simulink model "NewSim"  (R2016b)
settings: Solver=ode4  StartTime=0.0  StopTime=duration  FixedStep=t_step  RelTol=1e-3
values from neighbouring files (symbols this model uses):
  albedo = [0	0.367	0.12	0.15	0.06]'    [SimSetup.m]
  constants = [6.67408e-11; 299792458; 1361; 1.38064852e-23]    [SimSetup.m]
  Cyc_pos0 = Cyc_pos0*149597870.700e3    [SimSetup.m]
  Cyc_vel0 = Cyc_vel0*149597870.700e3/86400.0    [SimSetup.m]
  desired_trajectory = desired_trajectory*149597870.700e3    [SimSetup.m]
  dim = [6;30]    [SimSetup.m]
  emis = [0 0.9 0.9 0.8 0.93]'    [SimSetup.m]
  Ki = 1e-12    [SimSetup.m]
  Kp = 1e-3    (= 0.001)    [SimSetup.m]
  mass = [1.9885E+30	5.9722E+24	7.3490E+22	6.4171E+23	1.0800E+16,250000]'    [SimSetup.m]
  radii = [695700 6378.137 1737.53 3389.92 11.16666667]'    [SimSetup.m]
  SPM_pos0 = SPM_pos0*149597870.700e3    [SimSetup.m]
  SPM_vel0 = SPM_vel0*149597870.700e3/86400.0    [SimSetup.m]
  t_step = 60*10    (= 600)    [SimSetup.m]
  temp = [0 288 233 210 215]'    [SimSetup.m]
undefined symbols (not defined in the file or in its folder): getAccel, getTraj
settings Model: Creator=Jacob  LastModifiedBy=Jacob

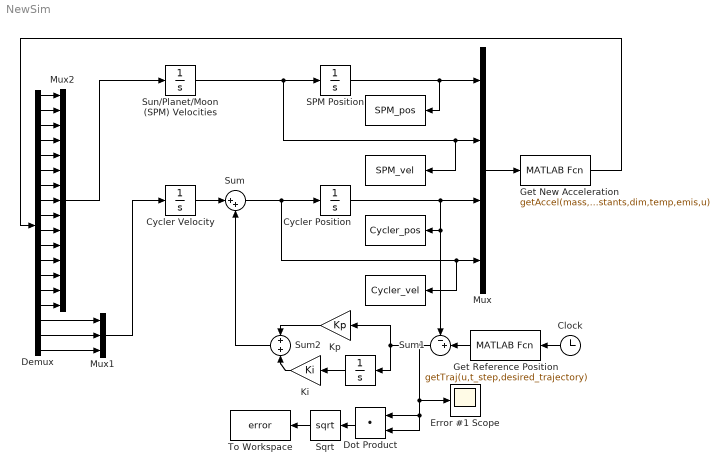
== system NewSim ==
  " " : ToWorkspace  VariableName=SPM_pos  SaveFormat=Timeseries  SampleTime=-1
  "  " : ToWorkspace  VariableName=SPM_vel  SaveFormat=Timeseries  SampleTime=-1
  "   " : ToWorkspace  VariableName=Cycler_pos  SaveFormat=Timeseries  SampleTime=-1
  "    " : ToWorkspace  VariableName=Cycler_vel  SaveFormat=Timeseries  SampleTime=-1
  "     " : Integrator  InitialCondition=[0,0,0]
  Clock : Clock
  Cycler Position : Integrator  InitialCondition=Cyc_pos0
  Cycler Velocity : Integrator  InitialCondition=Cyc_vel0
  Demux : Demux  Outputs=18
  Dot Product : DotProduct  InputSameDT=on  OutDataTypeStr=Inherit: Inherit via internal rule
  Error #1 Scope : Scope
  Get New Acceleration : MATLABFcn  MATLABFcn=getAccel(mass,albedo,radii,constants,dim,temp,emis,u)  OutputDimensions=18
  Get Reference Position : MATLABFcn  MATLABFcn=getTraj(u,t_step,desired_trajectory)  OutputDimensions=3
  Ki : Gain  Gain=Ki
  Kp : Gain  Gain=Kp
  Mux : Mux
  Mux1 : Mux  Inputs=3
  Mux2 : Mux  Inputs=15
  SPM Position : Integrator  InitialCondition=SPM_pos0
  Sqrt : Sqrt  SaturateOnIntegerOverflow=on
  Sum : Sum  Inputs=|++
  Sum1 : Sum  Inputs=-+|
  Sum2 : Sum
  Sun/Planet/Moon (SPM) Velocities : Integrator  InitialCondition=SPM_vel0
  To Workspace : ToWorkspace  VariableName=error  SaveFormat=Timeseries  SampleTime=-1
  wires:
  Sun/Planet/Moon (SPM) Velocities/1 -> "  "/1, Mux/2, SPM Position/1
  Mux/1 -> Get New Acceleration/1
  Demux/16 -> Mux1/1
  Demux/17 -> Mux1/2
  Demux/18 -> Mux1/3
  Demux/1 -> Mux2/1
  Demux/2 -> Mux2/2
  Demux/3 -> Mux2/3
  Demux/4 -> Mux2/4
  Demux/5 -> Mux2/5
  Demux/6 -> Mux2/6
  Demux/7 -> Mux2/7
  Demux/8 -> Mux2/8
  Demux/9 -> Mux2/9
  Demux/10 -> Mux2/10
  Demux/11 -> Mux2/11
  Demux/12 -> Mux2/12
  Demux/13 -> Mux2/13
  Demux/14 -> Mux2/14
  Demux/15 -> Mux2/15
  Mux2/1 -> Sun/Planet/Moon (SPM) Velocities/1
  Mux1/1 -> Cycler Velocity/1
  Cycler Velocity/1 -> Sum/1
  Sum/1 -> Cycler Position/1, "    "/1, Mux/4
  Get Reference Position/1 -> Sum1/2
  Clock/1 -> Get Reference Position/1
  Get New Acceleration/1 -> Demux/1
  Kp/1 -> Sum2/1
  Sum1/1 -> Error #1 Scope/1, Dot Product/2, Dot Product/1, "     "/1, Kp/1
  "     "/1 -> Ki/1
  Ki/1 -> Sum2/2
  Sum2/1 -> Sum/2
  SPM Position/1 -> Mux/1, " "/1
  Cycler Position/1 -> "   "/1, Sum1/1, Mux/3
  Dot Product/1 -> Sqrt/1
  Sqrt/1 -> To Workspace/1
